simulink model "realimentado"  (R2023b)
settings: Solver=VariableStepAuto  StartTime=0.0  StopTime=5  MaxStep=1e-5  RelTol=1e-3
values from neighbouring files (symbols this model uses):
  A = [0 1; 0 -p]    [realimentador.m]
  AccionDirecta = 0    [realimentador.m]
  B = [0; ke]    [realimentador.m]
  C = [1, 0]    [realimentador.m]
  consigna = 90    [realimentador.m]
  InicioEstimador = -100    [realimentador.m]
  ke = 7.3343e+03    (= 7334.3)    [realimentador.m]
  Ki = acker(Aamp, Bamp, [-0.5*p, -0.5*p, -0.7*p])    [realimentador.m]
  L = place(A', C', [-1.2*p, -1.3*p])'    [realimentador.m]
  p = s.yout{1}.Values.Data    [realimentador.m]
settings Model: Creator=erwinplanck  LastModifiedBy=erwinplanck

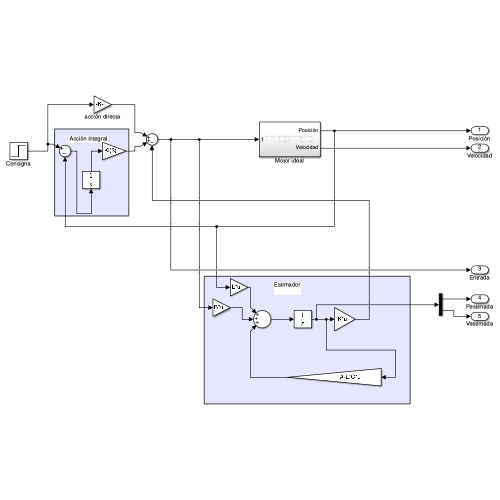
[thumbnail: Simulink's stored preview of the top-level diagram]
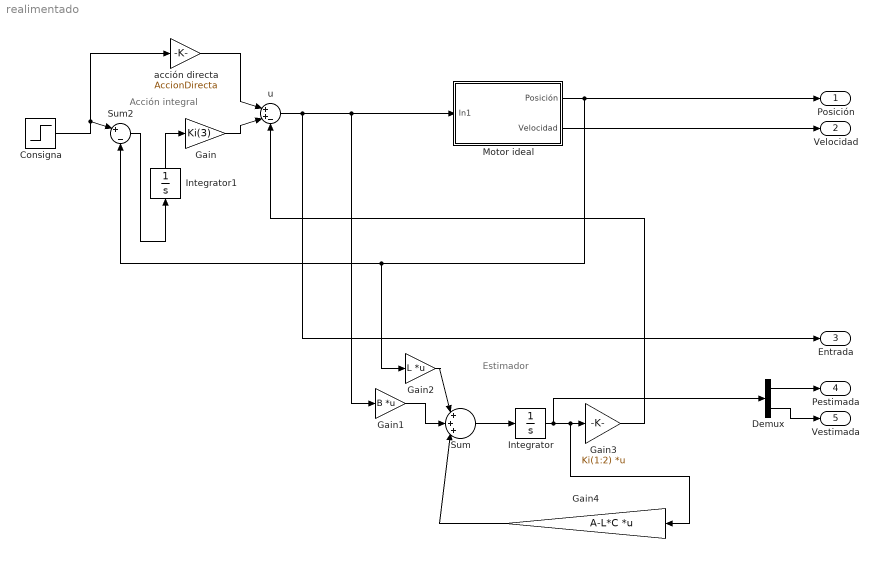
== system realimentado ==
  note: Acción integral
  note: Estimador
  Consigna : Step  Time=0  After=consigna  SampleTime=0
  Demux : Demux  Outputs=2
  Gain : Gain  Gain=Ki(3)
  Gain1 : Gain  Gain=B  Multiplication=Matrix(K*u)
  Gain2 : Gain  Gain=L  Multiplication=Matrix(K*u)
  Gain3 : Gain  Gain=Ki(1:2)  Multiplication=Matrix(K*u)
  Gain4 : Gain  Gain=A-L*C  Multiplication=Matrix(K*u)
  Integrator : Integrator  InitialCondition=InicioEstimador
  Integrator1 : Integrator
  Motor ideal : Subsystem
  Sum : Sum  Inputs=|+++|
  Sum2 : Sum  Inputs=|+|-
  acción directa : Gain  Gain=AccionDirecta
  u : Sum  Inputs=|++-
  Posición : Outport
  Velocidad : Outport  Port=2
  Entrada : Outport  Port=3
  Pestimada : Outport  Port=4
  Vestimada : Outport  Port=5
  wires:
  u/1 -> Entrada/1, Motor ideal/1(In1), Gain1/1
  Motor ideal/1(Posición) -> Posición/1, Sum2/2, Gain2/1
  Consigna/1 -> Sum2/1, acción directa/1
  acción directa/1 -> u/1
  Gain2/1 -> Sum/1
  Gain1/1 -> Sum/2
  Sum/1 -> Integrator/1
  Gain3/1 -> u/3
  Gain4/1 -> Sum/3
  Sum2/1 -> Integrator1/1
  Integrator1/1 -> Gain/1
  Gain/1 -> u/2
  Motor ideal/2(Velocidad) -> Velocidad/1
  Demux/1 -> Pestimada/1
  Demux/2 -> Vestimada/1
  Integrator/1 -> Demux/1, Gain4/1, Gain3/1

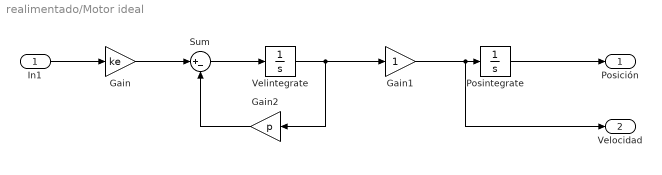
== system realimentado/Motor ideal ==
  In1 : Inport
  Gain : Gain  Gain=ke
  Gain1 : Gain
  Gain2 : Gain  Gain=p
  Posintegrate : Integrator
  Sum : Sum  Inputs=|+-
  Velintegrate : Integrator  InitialCondition=4
  Posición : Outport
  Velocidad : Outport  Port=2
  wires:
  Sum/1 -> Velintegrate/1
  Gain2/1 -> Sum/2
  Gain1/1 -> Velocidad/1, Posintegrate/1
  Posintegrate/1 -> Posición/1
  In1/1 -> Gain/1
  Velintegrate/1 -> Gain2/1, Gain1/1
  Gain/1 -> Sum/1
